simulink model "short_ct_test_1_ph_transformer"  (R2014b)
settings: Solver=ode23tb  StartTime=0.0  StopTime=5  MaxStep=1e-4  RelTol=1e-3
libraries: powerlib x5, powerlib_meascontrol x3
settings Model: Creator=Amr Saleh  LastModifiedBy=Amr Saleh

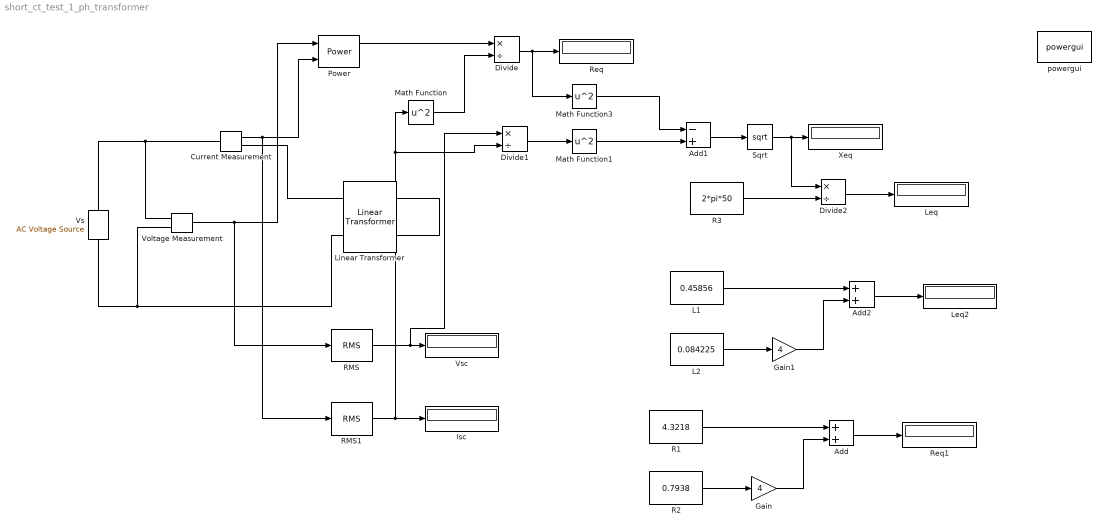
== system short_ct_test_1_ph_transformer ==
  Add : Sum
  Add1 : Sum  Inputs=-+
  Add2 : Sum
  Current Measurement : powerlib/Measurements/Current Measurement  PhasorSimulation=off  OutputType=Complex  PSBequivalent=0
  Divide : Product  Inputs=*/
  Divide1 : Product  Inputs=*/
  Divide2 : Product  Inputs=*/
  Gain : Gain  Gain=4
  Gain1 : Gain  Gain=4
  Isc : Display
  L1 : Constant  Value=0.45856
  L2 : Constant  Value=0.084225
  Leq : Display
  Leq2 : Display
  Linear Transformer : powerlib/Elements/Linear Transformer  UNITS=SI  NominalPower=[2000 50 ]  winding1=[220 4.3218 0.45856]  winding2=[110 0.7938 0.084225]  ThreeWindings=off  winding3=[3.15e+05 0.7938 0.084225]  RmLm=[1.0805e+06 2866]  Measurements=None  DataType=on
  Math Function : Math  Operator=square  SaturateOnIntegerOverflow=on
  Math Function1 : Math  Operator=square  SaturateOnIntegerOverflow=on
  Math Function3 : Math  Operator=square  SaturateOnIntegerOverflow=on
  Power : powerlib_meascontrol/Measurements/Power  Freq=50  Vinit=[1, 0]  Iinit=[1, 0]  Ts=0
  R1 : Constant  Value=4.3218
  R2 : Constant  Value=0.7938
  R3 : Constant  Value=2*pi*50
  RMS : powerlib_meascontrol/Measurements/RMS  TrueRMS=off  Freq=50  RMSInit=0  Ts=0
  RMS1 : powerlib_meascontrol/Measurements/RMS  TrueRMS=off  Freq=50  RMSInit=0  Ts=0
  Req : Display
  Req1 : Display
  Sqrt : Sqrt  SaturateOnIntegerOverflow=on
  Voltage Measurement : powerlib/Measurements/Voltage Measurement  PhasorSimulation=off  OutputType=Complex  PSBequivalent=0
  Vs : powerlib/Electrical Sources/AC Voltage Source  Amplitude=50*sqrt(2)  Phase=0  Frequency=50  SampleTime=0  Measurements=None
  Vsc : Display
  Xeq : Display
  powergui : powerlib/powergui  Priority=1  SimulationMode=Continuous  SolverType=Tustin/Backward Euler (TBE)  SampleTime=50e-6  frequency=60  SPID=off  DisableSnubberDevices=off  DisableRonSwitches=off  DisableVfSwitches=off  SwTol=0  DisplayEquations=off  Interpol=off  methode=off  Ts=100  frequencyindice=50  Pbase=100e6  ErrMax=1e-4  Iterations=50  UnitsV=kV  UnitsW=MW  FunctionMessages=off  echomessages=off  HookPort=off  EnableUseOfTLC=off  x0status=blocks  RestoreLinks=warning  ResistiveCurrentMeasurement=off  Frange=[0:2:500]  Ylog=off  Xlog=on  ShowGrid=off  save=off  variable=ZData  structure=0  ZoomFFT=off  StartTime=0.0  cycles=1  DisplayStyle=1  fundamental=60  FreqAxis=off  MaxFrequency=1000  frequencyindicesteady=1  RmsSteady=1  display=off
  wires:
  Voltage Measurement/1 -> Power/1, RMS/1
  Current Measurement/1 -> RMS1/1, Power/2
  RMS1/1 -> Divide1/2, Math Function/1, Isc/1
  Power/1 -> Divide/1
  Math Function/1 -> Divide/2
  Divide/1 -> Math Function3/1, Req/1
  RMS/1 -> Divide1/1, Vsc/1
  Divide1/1 -> Math Function1/1
  Math Function1/1 -> Add1/2
  Math Function3/1 -> Add1/1
  Add1/1 -> Sqrt/1
  Sqrt/1 -> Divide2/1, Xeq/1
  R3/1 -> Divide2/2
  Divide2/1 -> Leq/1
  R2/1 -> Gain/1
  R1/1 -> Add/1
  Gain/1 -> Add/2
  Add/1 -> Req1/1
  L2/1 -> Gain1/1
  L1/1 -> Add2/1
  Gain1/1 -> Add2/2
  Add2/1 -> Leq2/1
  connections:
  Vs/RConn1 -- Voltage Measurement/LConn1 -- Current Measurement/LConn1
  Current Measurement/RConn1 -- Linear Transformer/LConn1
  Linear Transformer/LConn2 -- Voltage Measurement/LConn2 -- Vs/LConn1
  Linear Transformer/RConn1 -- Linear Transformer/RConn2
